simulink model "GearShift_1650800352"  (R2021a)
settings: Solver=VariableStepAuto  StartTime=0.0  StopTime=100  RelTol=1e-3
undefined symbols (not defined in the file or in its folder): sigbuilder_block
settings Model: Creator=Ish  LastModifiedBy=Ish

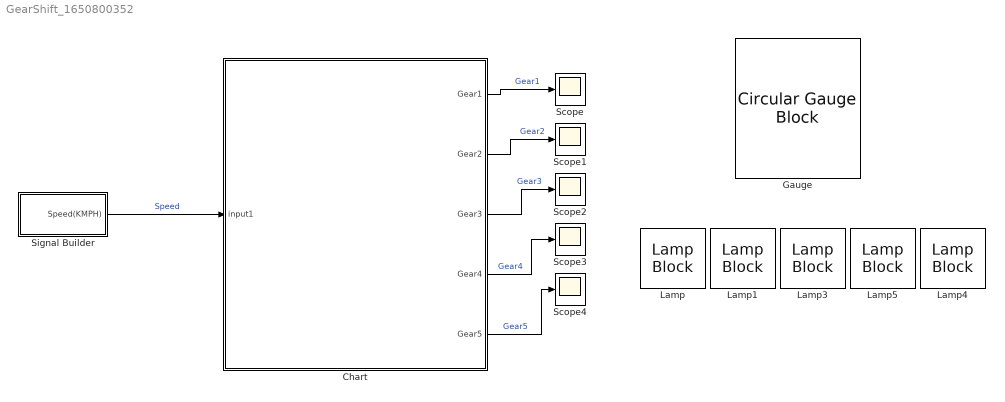
== system GearShift_1650800352 ==
  Chart : Stateflow chart  TreatAsAtomicUnit=on
  Gauge : CircularGaugeBlock
  Lamp{,1,3..5} (5 alike) : LampBlock
  Scope{,1..4} (5 alike) : Scope
  Signal Builder : Subsystem  Tag=STV Subsys  LoadFcn=sigbuilder_block('load');  StartFcn=sigbuilder_block('start');  StopFcn=sigbuilder_block('stop');  ClipboardFcn=sigbuilder_block('clipboard');  mask(Sigbuilder block){tuvar=[0:10]}
      mask help: Simulink:masks:SigbuilderBlock_MD
      mask init:
      | if ~strcmp(get_param(bdroot(gcbh),'SimulationStatus'),'stopped') tuvar = sigbuilder_block('maskInit'); end
      settings: CopyFcn=sigbuilder_block('copy');  DeleteFcn=sigbuilder_block('delete');  ModelCloseFcn=sigbuilder_block('modelClose');  PreSaveFcn=sigbuilder_block('preSave');  PauseFcn=sigbuilder_block('pause');  ContinueFcn=sigbuilder_block('continue');  NameChangeFcn=sigbuilder_block('namechange');  OpenFcn=sigbuilder_block('open',[153 156 544.5 355.5 ]);  CloseFcn=sigbuilder_block('close');
      mask Display: plot(0, 0, 100, 100,[2, 2, 32, 32, 2], [68, 8, 8, 68, 68],[32, 2], [38, 38], [32, 19, 2],[53, 60, 44], [32, 17, 17, 2],[16, 16, 31, 31]);txt = getActiveGroup(gcbh);text(2, 100, txt,'verticalAlignment', 'top');
  wires:
  Chart/1(Gear1) -> Scope/1  "Gear1"
  Chart/2(Gear2) -> Scope1/1  "Gear2"
  Chart/3(Gear3) -> Scope2/1  "Gear3"
  Chart/4(Gear4) -> Scope3/1  "Gear4"
  Chart/5(Gear5) -> Scope4/1  "Gear5"
  Signal Builder/1(Speed(KMPH)) -> Chart/1(input1)  "Speed"

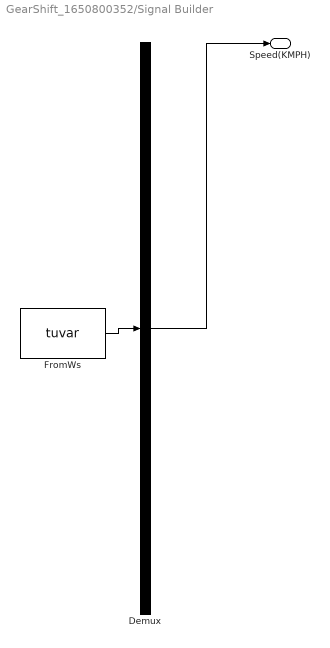
== system GearShift_1650800352/Signal Builder ==
  Demux : Demux  Tag=STV Demux  Outputs=1
      settings: DisplayOption=none
  FromWs : FromWorkspace  Tag=STV FromWs  VariableName=tuvar
      SigBuilderData=|
      | common.afterFinalStr = 'Extrapolate'
      | common.sampleTime = 0
      | dataSet.timeRange = [0 100]
      | dataSet.name = 'Sheet1'
      | sbobj.Groups.Name = 'Sheet1'
      | sbobj.Groups.Signals.Name = 'Speed(KMPH)'
      | sbobj.Groups.Signals.XData = [0 5 10 15 20 25 30 35 40 45 50 55 60 65 70 75 80 85 90 95 100]
      | sbobj.Groups.Signals.YData = [0 10 15 20 25 35 20 5 25 40 60 70 80 85 75 75 70 35 35 20 5]
      | sbobj.Groups.TimeRange = [0 100]
  Speed(KMPH) : Outport  Tag=STV Outport
  wires:
  Demux/1 -> Speed(KMPH)/1
  FromWs/1 -> Demux/1

== stateflow chart GearShift_1650800352/Chart ==
  state S1
    entry:Gear1=1
    exit:Gear1=0
  state S2
    entry:Gear2=1
    exit:Gear2=0
  state S3
    entry:Gear3=1
    exit:Gear3=0
  state S4
    entry:Gear4=1
    exit:Gear4=0
  state S5
    entry:Gear5=1
    exit:Gear5=0
  (default) -> S1
  S1 -> S2 : [input1>15]
  S2 -> S1 [order 2] : [input1<15]
  S2 -> S3 [order 1] : [input1>25]
  S3 -> S2 [order 2] : [input1<25]
  S3 -> S4 [order 1] : [input1>40]
  S4 -> S3 [order 2] : [input1<40]
  S4 -> S5 [order 1] : [input1>61]
  S5 -> S4 : [input1<61]
  data: Gear1 output; Gear2 output; Gear3 output; Gear4 output; Gear5 output; input1 input
